simulink model "flyrobot_test_kinematics"  (R2024a)
settings: Solver=VariableStepAuto  StartTime=0.0  StopTime=1  RelTol=1e-3
undefined symbols (not defined in the file): X, Y, Z
libraries: sm_lib x232, nesl_utility x21, robotcorelib x1
(part 1 of 6)
settings Model: Creator=73626  LastModifiedBy=HP

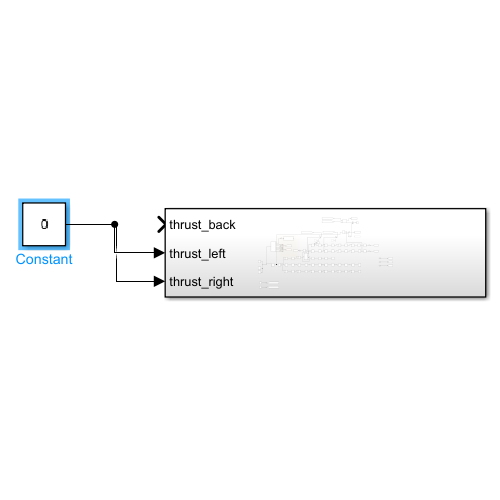
[thumbnail: Simulink's stored preview of the top-level diagram]
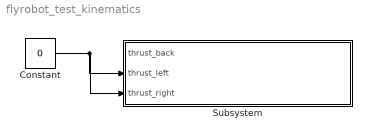
== system flyrobot_test_kinematics ==
  Constant : Constant  Value=0
  Subsystem : Subsystem
  wires:
  Constant/1 -> Subsystem/2(thrust_left), Subsystem/3(thrust_right)
